simulink model "eliminationofresistors"  (R2020b)
settings: Solver=VariableStepAuto  StartTime=0.0  StopTime=20  RelTol=1e-3
libraries: powerlib x13, simulink x1
settings Model: Creator=youss  LastModifiedBy=youss

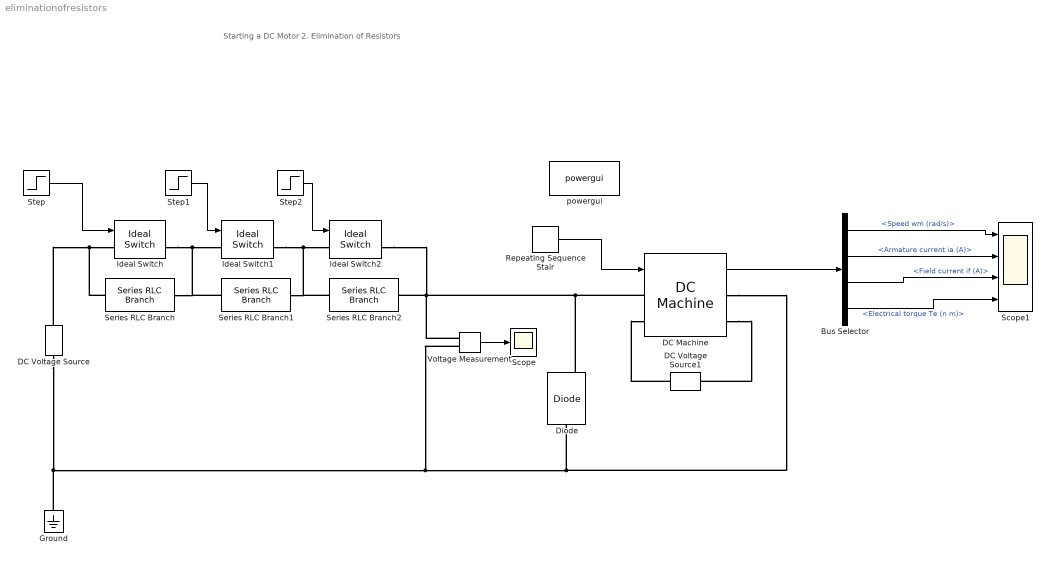
== system eliminationofresistors ==
  note: Starting a DC Motor
      | 2. Elimination of Resistors
  Bus Selector : BusSelector  OutputSignals=Speed wm (rad/s),Armature current ia (A),Field current if (A),Electrical torque Te (n m)
  DC Machine : powerlib/Machines/DC Machine  PresetModel=04: 10HP 240V 1750RPM Field:300V  MechanicalLoad=Torque TL  FieldType=Wound  ShowDetailedParameters=on  MeasurementBus=off  RLa=[1.086 0.01216]  RLf=[180 71.47]  Laf=0.6458  MachineConstant=Torque constant (N.m/A)  Ke=1.8  Kt=1.8  J=0.04251  Bm=0.003406  Tf=1.046  w0=1  Ifinit=0.666666666666667  TsPowergui=0  TsBlock=-1
  DC Voltage Source : powerlib/Electrical Sources/DC Voltage Source  Amplitude=240  Measurements=None
  DC Voltage Source1 : powerlib/Electrical Sources/DC Voltage Source  Amplitude=120  Measurements=None
  Diode : powerlib/Power Electronics/Diode  Ron=0.001  Lon=0  Vf=0.8  IC=0  UseSnubber=0  Rs=500  Cs=250e-9  Measurements=on
  Ground : powerlib/Elements/Ground  LConnTagsString=a
  Ideal Switch : powerlib/Power Electronics/Ideal Switch  Ron=0.001  Lon=0  IC=0  Rs=1e5  Cs=inf  Measurements=on
  Ideal Switch1 : powerlib/Power Electronics/Ideal Switch  Ron=0.001  Lon=0  IC=0  Rs=1e5  Cs=inf  Measurements=on
  Ideal Switch2 : powerlib/Power Electronics/Ideal Switch  Ron=0.001  Lon=0  IC=0  Rs=1e5  Cs=inf  Measurements=on
  Repeating Sequence Stair : simulink/Sources/Repeating Sequence Stair  OutValues=[0 3 ].'  tsamp=4  OutMin=[]  OutMax=[]  OutDataTypeStr=double  OutputDataTypeScalingMode=double  OutDataType=fixdt(0,8)  ConRadixGroup=Best Precision: Vector-wise  OutScaling=2^-12
  Scope : Scope
  Scope1 : Scope  NumInputPorts=4
  Series RLC Branch : powerlib/Elements/Series RLC Branch  LConnTagsString=__new0  RConnTagsString=__new0  BranchType=R  Resistance=12.5  Inductance=1e-3  SetiL0=off  InitialCurrent=0  Capacitance=1e-6  Setx0=off  InitialVoltage=0  Measurements=None
  Series RLC Branch1 : powerlib/Elements/Series RLC Branch  LConnTagsString=__new0  RConnTagsString=__new0  BranchType=R  Resistance=7.5  Inductance=1e-3  SetiL0=off  InitialCurrent=0  Capacitance=1e-6  Setx0=off  InitialVoltage=0  Measurements=None
  Series RLC Branch2 : powerlib/Elements/Series RLC Branch  LConnTagsString=__new0  RConnTagsString=__new0  BranchType=R  Resistance=2.5  Inductance=1e-3  SetiL0=off  InitialCurrent=0  Capacitance=1e-6  Setx0=off  InitialVoltage=0  Measurements=None
  Step : Step  SampleTime=2
  Step1 : Step  SampleTime=4
  Step2 : Step  SampleTime=5
  Voltage Measurement : powerlib/Measurements/Voltage Measurement  PhasorSimulation=off  OutputType=Complex  PSBequivalent=0
  powergui : powerlib/powergui  Priority=1  SimulationMode=Discrete  SampleTime=0.0001  frequency=60  Iterations=50  frequencyindice=0  Pbase=100e6  ErrMax=1e-4  UnitsV=kV  UnitsW=MW  buscounter=0  FunctionMessages=off  echomessages=off  EnableUseOfTLC=off  CurrentSourceSwitches=off  DisableSnubberDevices=off  DisableRonSwitches=off  DisableVfSwitches=off  DisplayEquations=off  AutomaticDiscreteSolvers=off  SolverType=Tustin/Backward Euler (TBE)  Interpol=off  ExternalGateDelay=off  methode=off  Ts=100  x0status=blocks  SPID=on  SwTol=0  HookPort=off  NonlinearTolerance=1e-4  nMaxIteration=100  ContinueOnMaxIteration=off  RestoreLinks=warning  ResistiveCurrentMeasurement=off  Frange=[0:2:500]  Ylog=off  Xlog=on  ShowGrid=off  save=off  variable=ZData  structure=0  ZoomFFT=off  StartTime=0.0  cycles=1  DisplayStyle=1  fundamental=60  FreqAxis=off  MaxFrequency=1000  frequencyindicesteady=1  RmsSteady=1  display=off
  wires:
  Step/1 -> Ideal Switch/1
  Step1/1 -> Ideal Switch1/1
  Step2/1 -> Ideal Switch2/1
  Voltage Measurement/1 -> Scope/1
  Repeating Sequence Stair/1 -> DC Machine/1
  DC Machine/1 -> Bus Selector/1
  Bus Selector/1 -> Scope1/1  "<Speed wm (rad/s)>"
  Bus Selector/2 -> Scope1/2  "<Armature current ia (A)>"
  Bus Selector/3 -> Scope1/3  "<Field current if (A)>"
  Bus Selector/4 -> Scope1/4  "<Electrical torque Te (n m)>"
  connections:
  DC Voltage Source/RConn1 -- Series RLC Branch/LConn1 -- Ideal Switch/LConn1
  Ideal Switch/RConn1 -- Series RLC Branch/RConn1 -- Series RLC Branch1/LConn1 -- Ideal Switch1/LConn1
  Ideal Switch1/RConn1 -- Series RLC Branch2/LConn1 -- Series RLC Branch1/RConn1 -- Ideal Switch2/LConn1
  DC Machine/LConn1 -- Voltage Measurement/LConn1 -- Ideal Switch2/RConn1 -- Series RLC Branch2/RConn1 -- Diode/RConn1
  DC Voltage Source/LConn1 -- Ground/LConn1 -- Voltage Measurement/LConn2 -- DC Machine/RConn1 -- Diode/LConn1
  DC Voltage Source1/RConn1 -- DC Machine/LConn2
  DC Machine/RConn2 -- DC Voltage Source1/LConn1
